simulink model "PI_Controller"  (R2020a)
settings: Solver=ode23s  StartTime=0.0  StopTime=0.1  MaxStep=0.001  RelTol=1e-3
undefined symbols (not defined in the file): kd, ki, kp, n
settings Model: DataDictionary=Ques_4_Parameters.sldd  Creator=DELL  LastModifiedBy=DELL
settings DataIOCC: SaveOutput=off  SaveTime=off

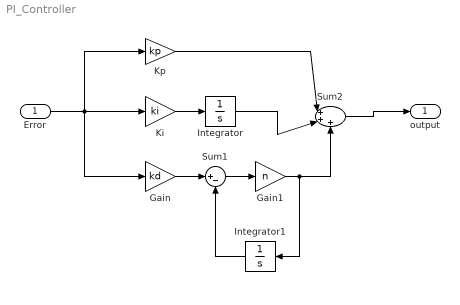
== system PI_Controller ==
  Error : Inport  OutDataTypeStr=double  PortDimensions=1  SampleTime=0
  Gain : Gain  Gain=kd
  Gain1 : Gain  Gain=n
  Integrator : Integrator
  Integrator1 : Integrator
  Ki : Gain  Gain=ki
  Kp : Gain  Gain=kp
  Sum1 : Sum  Inputs=|+-
  Sum2 : Sum  Inputs=|+++
  output : Outport  OutDataTypeStr=double  PortDimensions=1  SampleTime=0
  wires:
  Kp/1 -> Sum2/1
  Sum2/1 -> output/1
  Ki/1 -> Integrator/1
  Sum1/1 -> Gain1/1
  Gain1/1 -> Sum2/3, Integrator1/1
  Error/1 -> Kp/1, Ki/1, Gain/1
  Integrator/1 -> Sum2/2
  Integrator1/1 -> Sum1/2
  Gain/1 -> Sum1/1
